simulink model "attractor_reconstruction"  (R2019b)
settings: Solver=FixedStepAuto  StartTime=0.0  StopTime=10.0  RelTol=1e-3
settings Model: Creator=zuga_  LastModifiedBy=zuga_

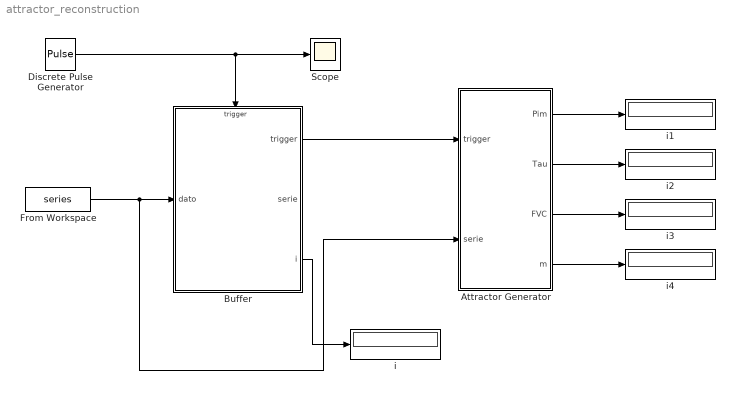
== system attractor_reconstruction ==
  Attractor Generator : Stateflow chart  BlockKeywords=__PRM__SERIALIZED__DATA__:Stateflow Chart,Stateflow Diagram  TreatAsAtomicUnit=on
  Buffer : Stateflow chart  BlockKeywords=__PRM__SERIALIZED__DATA__:Stateflow Chart,Stateflow Diagram  TreatAsAtomicUnit=on
  Discrete Pulse Generator : DiscretePulseGenerator  PulseType=Time based  Period=1/173.62  PulseWidth=50
  From Workspace : FromWorkspace  VariableName=series  SampleTime=0
  Scope : Scope
  i{,1..4} (5 alike) : Display
  wires:
  Discrete Pulse Generator/1 -> Scope/1, Buffer/Trigger
  Buffer/3(i) -> i/1
  Buffer/1(trigger) -> Attractor Generator/1(trigger)
  From Workspace/1 -> Attractor Generator/2(serie), Buffer/1(dato)
  Attractor Generator/1(Pim) -> i1/1
  Attractor Generator/2(Tau) -> i2/1
  Attractor Generator/3(FVC) -> i3/1
  Attractor Generator/4(m) -> i4/1

== stateflow chart attractor_reconstruction/Buffer ==
  state AddData
    %en: serie = buffer(serie, i, dato);
    en: i = i+1;
  state Accelerate
    en: trigger = true;
  state End2
    en: trigger = false;
  (default) -> AddData : {
      | trigger = false;
      | size = 64;
      | serie = zeros(size, 1);
      | i = 1;
      | }
  AddData -> AddData [order 1] : [i < size]
  AddData -> Accelerate [order 2]
  Accelerate -> End2
  data: serie_in function_input; index function_input; data function_input; serie_out function_output; dato input double; trigger output boolean; serie output double size=5000; i output double; size local double
  events: event input RISING_EDGE_EVENT
  function serie_out = buffer(serie_in, index, data):
    | function serie_out = buffer(serie_in, index, data)
    |     if index == 1
    |         serie_out = data(((index-1)*64)+1:index*64-1);
    |     else
    |        serie_out = [serie_in data(((index-1)*64)+1:index*64-1)];
    |     end
    | end

== stateflow chart attractor_reconstruction/Attractor Generator ==
  (default) -> (junction 15) : {flag = false;}
  (junction 15) -> (junction 16) [order 1] : [flag == false && trigger == true]
  (junction 15) -> (junction 17) [order 2]
  (junction 16) -> (junction 18) : {
      | [Pim, Tau] = pim(serie, 64, 64);
      | [FVC, m] = knn_deneme(serie, Tau, 64, 15, 2);
      | flag = false;
      | }
  (junction 18) -> (junction 17)
  (junction 17) -> (junction 23)
  data: x function_input; taumax function_input; particiones function_input; PIM function_output; Optau function_output; x function_input; Optau function_input; mmax function_input; rtol function_input; atol function_input; FNN function_output; emb_dim function_output; Pim output double size=[1,120000]; Tau output double; FVC output double; m output double size=1; flag local boolean; trigger input boolean; serie input double
  function [PIM,Optau] = pim(x, taumax, particiones):
    | % [PIM,Optau] = pim(x, taumax, particiones)
    | % e.g.taumax = 64; particiones = 128;
    | % Devuelve la grafica de I(x_n,x_{n + Tau})
    | % y el valor optimo de retraso
    | function [PIM,Optau] = pim(x, taumax, particiones)
    |   % Normalizacion de la x
    |   x = (x - min(x))/(max(x) - min(x));
    |   N = length(x);
    |   AMI = ami(x, 1:taumax, particiones, N);
    |   PIM = zeros(size(AMI));
    |   PIM = AMI;
    |   if primin(PIM,N) == 0
    |     Optau = taumax;
    |   else
    |     Optau = primin(PIM,N);
    |   end
    |   figure
    |   plot(0:length(PIM) - 1,PIM);
    |   title('Mutual information and time delay')
    |   ylabel('Mutual information')
    |   xlabel('Time delay')
    | 
    |   % disp(Optau)
    | end
    | 
    | 
    | function mutua = ami(x,tau,k,N)
    |   % mutua = zeros(length(tau), 1);
    |   mutua = [];
    |   % I(x_n,x_{n + \tau}) = pim(x, tau, K, Histograma)
    |   for i = 1:length(tau)
    |     for k1 = 1:k
    |       for k2 = 1:k
    |       % Histogramas unidimensionales
    |       px = find((k1 - 1)/k<x(1:N - tau(i)) & x(1:N - tau(i))<= k1/k);
    |       py = find((k2 - 1)/k<x(1 + tau(i):N) & x(1 + tau(i):N)<= k2/k);
    |       % Histograma bidimensional
    |       Ixy = find((k1 - 1)/k<x(1:N - tau(i)) & x(1:N - tau(i))<= k1/k & ...
    |                     (k2-1)/k<x(1 + tau(i):N) & x(1 + tau(i):N)<= k2/k);
    |       Ixy = length(Ixy);
    |       Pxy = Ixy;
    |       % Densidades de probabilidad
    |       if Pxy > 0
    |         Px = length(px)/(N-tau(i));
    |         Py = length(py)/(N-tau(i));
    |         Pxy = Pxy/(N-tau(i));
    |         % Promedio de informacion mutua
    |         % mutua(i) = mutua(i) + Pxy*log2(Pxy/px/py);
    |         mutua = [mutua, Pxy*log2(Pxy/(Px*Py))];
    |       end
    |       end
    |     end
    |   end
    | end
    | 
    | 
    | function T = primin(X,N)
    |   % Devuelve el primer minimo de I(x_n,x_{n + T})
    |   % j = 0;
    |   T = 0;
    |   derivp1 = zeros(N-3,1);
    |   derivp2 = derivp1;
    |   for m = 3:N
    |     derivp1(m-2) = X(m-1)-X(m-2);
    |     derivp2(m-2) = X(m)-X(m-1);
    |     if (derivp1(m-2)<0)&&(derivp2(m-2)>0)
    |       % j = j + 1;
    |       T = m-2;
    |       break
    |     end
    |   end
    | end
  function [FNN, emb_dim] = knn_deneme(x, Optau, mmax, rtol, atol):
    | function [FNN, emb_dim] = knn_deneme(x, Optau, mmax, rtol, atol)
    |   % x: time series
    |   % Optau: time delay
    |   % mmax: maximum embedding dimension
    |   % reference: M.B.Kennel, R.Brown, and H.D.I. Abarbanel,
    |   % Determining embedding dimension for phase-space reconstruction
    |   % using a geometrical construction, Phys. Rev. A 45, 3403 (1992).
    |   % modified by: Walther Carballo Hernández (2015)
    | 
    |   % rtol = 15
    |   % atol = 2;
    |   N = length(x);
    |   % Standard deviation
    |   Ra = std(x, 1);
    |   emb_dim = 0;
    |   FNN = zeros(mmax, 1);
    | 
    |   % Compute the FNN with each m iteration
    |   for m = 1:mmax
    |     M = N-m*Optau;
    |     % Reconstruct the attractor
    |     Y = psr_deneme(x, m, Optau, M);
    |     FNN(m, 1) = 0;
    |     % Each iteration calculates the distance from one point
    |     % in the attractor with other point in the space state
    |     for n = 1:M
    |       y0 = ones(M, 1)*Y(n, :);
    |       % Obtaining the distance vector
    |       distance = sqrt(sum((Y-y0).^2,2));
    |       % Sorting the distance vector
    |       [neardis nearpos] = sort(distance);
    |       % Obtaining absolut evalue
    |       D = abs(x(n + m*Optau) - x(nearpos(2) + m*Optau));
    |       % Obtaining square root
    |       R = sqrt(D.^2 + neardis(2).^2);
    |       if (D/neardis(2) > rtol || R/Ra > atol)
    |         FNN(m,1) = FNN(m,1) + 1;
    |       end
    |     end
    |     if (FNN(m,1) / FNN(1,1))*100<0.01
    |       emb_dim = m;
    |       break
    |     end
    |   end
    |   % Calculating embedding dimension
    |   if emb_dim == 0
    |     min_indexes = find(FNN(:, 1) == min(FNN(:,1)));
    |     emb_dim = min_indexes(1, 1);
    |   end
    |   % Percentage of the FNN
    |   FNN = (FNN./FNN(1,1))*100;
    |   % Plot results
    |   figure
    |   plot(1:length(FNN), FNN)
    |   title('Minimum embedding dimension with false nearest neighbours')
    |   xlabel('Embedding dimension')
    |   ylabel('The percentage of false nearest neighbours')
    | end
